simulink model "Experiment1_simulink"  (R2021a)
settings: Solver=VariableStepAuto  StartTime=0.0  StopTime=0.1  RelTol=1e-3
libraries: dspfdesign x1
settings Model: Creator=Dell  LastModifiedBy=Dell

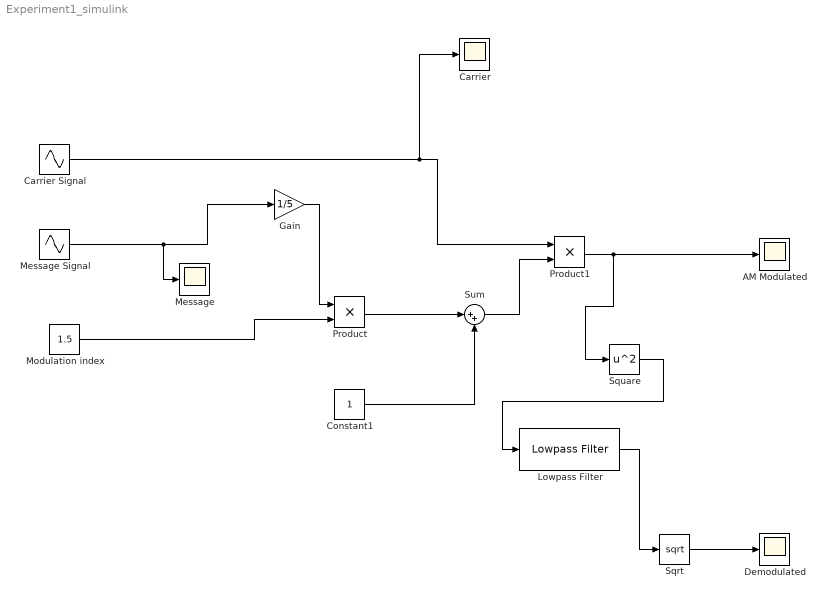
== system Experiment1_simulink ==
  AM Modulated : Scope
  Carrier : Scope
  Carrier Signal : Sin  Amplitude=5/1.5  Frequency=2*pi*10000  SampleTime=1e-6
  Constant1 : Constant
  Demodulated : Scope
  Gain : Gain  Gain=1/5
  Lowpass Filter : dspfdesign/Lowpass Filter  FilterType=FIR  DesignForMinimumOrder=on  FilterOrder=50  PassbandFrequency=500  StopbandFrequency=3000  PassbandRipple=0.1  StopbandAttenuation=80  InheritSampleRate=on  SampleRate=44100  SimulateUsing=Interpreted execution  roundingMode=Floor  coeffsDataTypeStr=fixdt(1,16)
  Message : Scope
  Message Signal : Sin  Amplitude=5  Frequency=2*pi*100  SampleTime=1e-6
  Modulation index : Constant  Value=1.5
  Product : Product
  Product1 : Product
  Sqrt : Sqrt  SaturateOnIntegerOverflow=on
  Square : Math  Operator=square  SaturateOnIntegerOverflow=on
  Sum : Sum  Inputs=|++
  wires:
  Modulation index/1 -> Product/2
  Message Signal/1 -> Message/1, Gain/1
  Constant1/1 -> Sum/2
  Product/1 -> Sum/1
  Sum/1 -> Product1/2
  Gain/1 -> Product/1
  Square/1 -> Lowpass Filter/1
  Lowpass Filter/1 -> Sqrt/1
  Sqrt/1 -> Demodulated/1
  Product1/1 -> Square/1, AM Modulated/1
  Carrier Signal/1 -> Carrier/1, Product1/1
